simulink library "Pitch_Functions"  (Simulink 6.5)
undefined symbols (not defined in the file or in its folder): A, ABS, B, C, D, P_PitchProfilerAccLim, P_PitchProfilerMaxGain, P_PitchProfilerPostDelay, P_PitchProfilerPreDelay, P_PitchProfilerSpdLim, P_PitchProfilerTc, P_PitchProfilerTcRatio, P_PitchSpinningPos, PITCH_CYCLE_TIME, RND, SQR
libraries: StandardLib x187, WindLib x15, Pitch_Functions x6, simulink x4
(part 1 of 3)
settings Model: Creator=200011716  LastModifiedBy=jschwein

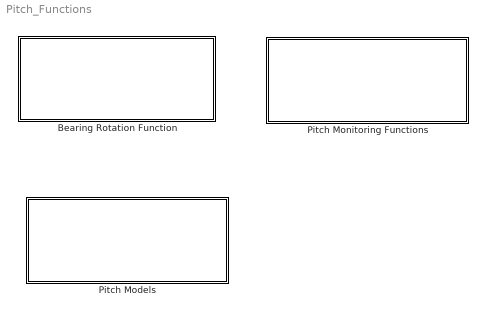
== system Pitch_Functions ==
  Bearing Rotation Function : Subsystem
      mask Display: disp('Bearing Rotation Function (BRF)')
  Pitch Models : Subsystem
      mask Display: disp('Pitch Models')
  Pitch Monitoring Functions : Subsystem
      mask Display: disp('Pitch Monitoring Functions')

== system Pitch_Functions/Bearing Rotation Function ==
  USRB_BladeAtLimSwtchLessthanRef : Subsystem  TreatAsAtomicUnit=on
      settings: MinAlgLoopOccurrences=on
  USRB_BladeAtReferenceDetect : Subsystem  TreatAsAtomicUnit=on
      settings: MinAlgLoopOccurrences=on
  USRB_BladeCompleted : Subsystem  TreatAsAtomicUnit=on
      settings: MinAlgLoopOccurrences=on
  USRB_LimitSwitchPickedUp : Subsystem  TreatAsAtomicUnit=on
      settings: MinAlgLoopOccurrences=on
  USRB_LimitSwitchPickedUpTrail : Subsystem  TreatAsAtomicUnit=on
      settings: MinAlgLoopOccurrences=on
  USRB_StartBladeMotionCmd : Subsystem  TreatAsAtomicUnit=on
      settings: MinAlgLoopOccurrences=on

== system Pitch_Functions/Pitch Models ==
  USRB_PitchProfiler : Subsystem  TreatAsAtomicUnit=on
      settings: MinAlgLoopOccurrences=on

== system Pitch_Functions/Pitch Monitoring Functions ==
  USRB_PitchProfilers : Subsystem  TreatAsAtomicUnit=on
      settings: MinAlgLoopOccurrences=on
  USRB_Pitch_AxisState1 : Subsystem  TreatAsAtomicUnit=on
  USRB_Pitch_BladeImplausible : Subsystem  TreatAsAtomicUnit=on
  USRB_Pitch_BladePitching : Subsystem  TreatAsAtomicUnit=on
  USRB_Pitch_Status : Subsystem  TreatAsAtomicUnit=on
  USRB_SevereBladeProblem : Subsystem  TreatAsAtomicUnit=on
  USRB_TransDelay : Subsystem  TreatAsAtomicUnit=on

== system Pitch_Functions/Bearing Rotation Function/USRB_BladeAtLimSwtchLessthanRef ==
  Limit89Switch : Inport  DataType=boolean
  PitchActual : Inport  Port=2  DataType=single
  Ref : Inport  Port=3  DataType=single
  AND : StandardLib/Logical operations/AND  RepeatCnt=1  SampleTime=-1  ExecutionOrder=0
  Constant : Constant  Value=1  OutDataTypeMode=boolean  OutDataType=sfix(16)  ConRadixGroup=Use specified scaling  OutScaling=2^0  SampleTime=inf  FramePeriod=inf
  Constant1 : Constant  Value=0  OutDataTypeMode=single  OutDataType=sfix(16)  ConRadixGroup=Use specified scaling  OutScaling=2^0  SampleTime=inf  FramePeriod=inf
  LT : StandardLib/Math operations/LT  Equation=<  DataType=SINGLE  SampleTime=-1  ExecutionOrder=0
  MOVE : StandardLib/Memory operations/MOVE  DataType=BOOLEAN  SampleTime=-1  ExecutionOrder=0
  BladeAt89 : Outport  DataType=boolean
  wires:
  Constant1/1 -> LT/3
  Constant/1 -> MOVE/2
  Ref/1 -> LT/2
  MOVE/1 -> AND/1
  LT/1 -> AND/2
  PitchActual/1 -> LT/1
  Limit89Switch/1 -> MOVE/1
  AND/1 -> BladeAt89/1

== system Pitch_Functions/Bearing Rotation Function/USRB_BladeAtReferenceDetect ==
  PitchActual : Inport  DataType=single
  Reference : Inport  Port=2  DataType=single
  PitchSpeed : Inport  Port=3  DataType=single
  PositionSensitivity : Inport  Port=4  DataType=single
  SpeedSensitivity : Inport  Port=5  DataType=single
  FeatherState : Inport  Port=6  DataType=boolean
  AND : StandardLib/Logical operations/AND  RepeatCnt=2  SampleTime=-1  ExecutionOrder=0
  Constant : Constant  Value=0  OutDataTypeMode=single  OutDataType=sfix(16)  ConRadixGroup=Use specified scaling  OutScaling=2^0  SampleTime=inf  FramePeriod=inf
  Constant1 : Constant  Value=0  OutDataTypeMode=single  OutDataType=sfix(16)  ConRadixGroup=Use specified scaling  OutScaling=2^0  SampleTime=inf  FramePeriod=inf
  Constant2 : Constant  Value=0  OutDataTypeMode=single  OutDataType=sfix(16)  ConRadixGroup=Use specified scaling  OutScaling=2^0  SampleTime=inf  FramePeriod=inf
  EQ : StandardLib/Math operations/EQ  Equation===  DataType=SINGLE  SampleTime=-1  ExecutionOrder=0
  EQ1 : StandardLib/Math operations/EQ  Equation===  DataType=SINGLE  SampleTime=-1  ExecutionOrder=0
  BladeAtRef : Outport  DataType=boolean
  wires:
  PitchActual/1 -> EQ/1
  Reference/1 -> EQ/2
  Constant/1 -> EQ/3
  PositionSensitivity/1 -> EQ/4
  PitchSpeed/1 -> EQ1/1
  Constant1/1 -> EQ1/2
  Constant2/1 -> EQ1/3
  SpeedSensitivity/1 -> EQ1/4
  EQ/1 -> AND/1
  EQ1/1 -> AND/2
  AND/1 -> BladeAtRef/1
  FeatherState/1 -> AND/3

== system Pitch_Functions/Bearing Rotation Function/USRB_BladeCompleted ==
  PitchComplete : Inport  DataType=boolean
  PitchActive : Inport  Port=2  DataType=boolean
  BladeAt89 : Inport  Port=3  DataType=boolean
  BRFComplete : Inport  Port=4  DataType=boolean
  ManualReset : Inport  Port=5  DataType=boolean
  LimitSwitch94PickedUp : Inport  Port=6  DataType=boolean
  TooLong : Inport  Port=7  DataType=boolean
  ExtendedPause : Inport  Port=8  DataType=boolean
  Abort : Inport  Port=9  DataType=boolean
  AND : StandardLib/Logical operations/AND  RepeatCnt=1  SampleTime=-1  ExecutionOrder=0
  AND1 : StandardLib/Logical operations/AND  RepeatCnt=1  SampleTime=-1  ExecutionOrder=0
  Constant : Constant  Value=1  OutDataTypeMode=boolean  OutDataType=sfix(16)  ConRadixGroup=Use specified scaling  OutScaling=2^0  SampleTime=inf  FramePeriod=inf
  LATCH : StandardLib/Logical operations/LATCH  SampleTime=-1  ExecutionOrder=0
  OR : StandardLib/Logical operations/OR  RepeatCnt=1  SampleTime=-1  ExecutionOrder=0
  OR1 : StandardLib/Logical operations/OR  RepeatCnt=4  SampleTime=-1  ExecutionOrder=0
  Terminator : Terminator
  BladeComplete : Outport  DataType=boolean
  wires:
  Abort/1 -> OR1/5
  ExtendedPause/1 -> OR1/4
  TooLong/1 -> OR1/3
  PitchActive/1 -> AND/2
  PitchComplete/1 -> AND/1
  Constant/1 -> LATCH/3
  ManualReset/1 -> OR1/2
  BRFComplete/1 -> OR1/1
  OR1/1 -> LATCH/2
  LATCH/2 -> Terminator/1
  LATCH/1 -> BladeComplete/1
  AND1/1 -> OR/2
  BladeAt89/1 -> AND1/1
  OR/1 -> LATCH/1
  LimitSwitch94PickedUp/1 -> AND1/2
  AND/1 -> OR/1

== system Pitch_Functions/Bearing Rotation Function/USRB_LimitSwitchPickedUp ==
  BladeActive : Inport  DataType=boolean
  Limit94Switch1 : Inport  Port=2  DataType=boolean
  Complete : Inport  Port=3  DataType=boolean
  AND : StandardLib/Logical operations/AND  RepeatCnt=1  SampleTime=-1  ExecutionOrder=0
  Constant10 : Constant  Value=1  OutDataTypeMode=boolean  OutDataType=sfix(16)  ConRadixGroup=Use specified scaling  OutScaling=2^0  SampleTime=inf  FramePeriod=inf
  LATCH : StandardLib/Logical operations/LATCH  SampleTime=-1  ExecutionOrder=0
  Terminator12 : Terminator
  LimitSwitchPickedUp : Outport  DataType=boolean
  wires:
  BladeActive/1 -> AND/1
  Limit94Switch1/1 -> AND/2
  AND/1 -> LATCH/1
  Complete/1 -> LATCH/2
  LATCH/1 -> LimitSwitchPickedUp/1
  LATCH/2 -> Terminator12/1
  Constant10/1 -> LATCH/3

== system Pitch_Functions/Bearing Rotation Function/USRB_LimitSwitchPickedUpTrail ==
  BladeActive : Inport  DataType=boolean
  Limit94Switch1 : Inport  Port=2  DataType=boolean
  Complete : Inport  Port=3  DataType=boolean
  AND : StandardLib/Logical operations/AND  RepeatCnt=1  SampleTime=-1  ExecutionOrder=0
  Constant1 : Constant  Value=0  OutDataTypeMode=uint32  OutDataType=sfix(16)  ConRadixGroup=Use specified scaling  OutScaling=2^0  SampleTime=inf  FramePeriod=inf
  Constant10 : Constant  Value=1  OutDataTypeMode=boolean  OutDataType=sfix(16)  ConRadixGroup=Use specified scaling  OutScaling=2^0  SampleTime=inf  FramePeriod=inf
  LATCH : StandardLib/Logical operations/LATCH  SampleTime=-1  ExecutionOrder=0
  NOT : StandardLib/Logical operations/NOT  SampleTime=-1  ExecutionOrder=0
  PULSE1 : StandardLib/Sequencing/PULSE  SampleTime=-1  ExecutionOrder=0
  Terminator{12,14..19} (7 alike) : Terminator
  LimitSwitchPickedUp : Outport  DataType=boolean
  wires:
  PULSE1/1 -> AND/2
  NOT/2 -> PULSE1/1
  Constant1/1 -> PULSE1/2
  PULSE1/6 -> Terminator18/1
  PULSE1/5 -> Terminator17/1
  PULSE1/4 -> Terminator16/1
  PULSE1/3 -> Terminator15/1
  PULSE1/2 -> Terminator14/1
  NOT/1 -> Terminator19/1
  Constant10/1 -> LATCH/3
  LATCH/2 -> Terminator12/1
  LATCH/1 -> LimitSwitchPickedUp/1
  Complete/1 -> LATCH/2
  AND/1 -> LATCH/1
  Limit94Switch1/1 -> NOT/1
  BladeActive/1 -> AND/1

== system Pitch_Functions/Bearing Rotation Function/USRB_StartBladeMotionCmd ==
  Blade_to_Index : Inport  DataType=int16
  bladenum : Inport  Port=2  DataType=int16
  StartCondition : Inport  Port=3  DataType=boolean
  AND : StandardLib/Logical operations/AND  RepeatCnt=1  SampleTime=-1  ExecutionOrder=0
  Constant : Constant  Value=0  OutDataTypeMode=int16  OutDataType=sfix(16)  ConRadixGroup=Use specified scaling  OutScaling=2^0  SampleTime=inf  FramePeriod=inf
  Constant1 : Constant  Value=10000  OutDataTypeMode=uint32  OutDataType=sfix(16)  ConRadixGroup=Use specified scaling  OutScaling=2^0  SampleTime=inf  FramePeriod=inf
  EQ : StandardLib/Math operations/EQ  Equation===  DataType=INT16  SampleTime=-1  ExecutionOrder=0
  PULSE : StandardLib/Sequencing/PULSE  SampleTime=-1  ExecutionOrder=0
  Terminator{,1..4} (5 alike) : Terminator
  StartBlade : Outport  DataType=boolean
  wires:
  Constant1/1 -> PULSE/2
  PULSE/6 -> Terminator4/1
  PULSE/5 -> Terminator3/1
  PULSE/4 -> Terminator2/1
  PULSE/3 -> Terminator1/1
  PULSE/2 -> Terminator/1
  PULSE/1 -> StartBlade/1
  StartCondition/1 -> AND/2
  AND/1 -> PULSE/1
  bladenum/1 -> EQ/2
  Blade_to_Index/1 -> EQ/1
  EQ/1 -> AND/1
  Constant/1 -> EQ/4, EQ/3

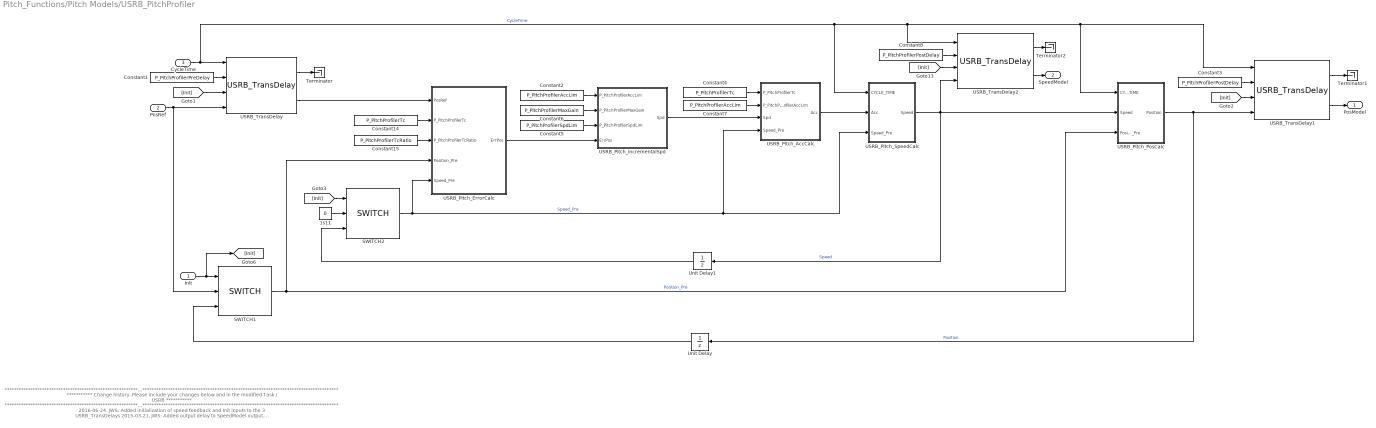
== system Pitch_Functions/Pitch Models/USRB_PitchProfiler ==
  note: ***********************************************************************************************************************************************
      | ***********         Change history. Please include your changes below and in the modified Task / USRB         ***********
      | ***********************************************************************************************************************************************
      | 2016-06-24, JWS: Added initialization of speed feedback and Init inputs to the 3 USRB_TransDelays
      | 2015-03-21, JWS: Added output delay to SpeedModel output.
      | 2015-11-04, JWS: Updated USRB name.
      | 2015-09-11, JWS: Replaced constant blocks with inputs.  Added SpeedModel output.
      | ***********************************************************************************************************************************************
  Init : Inport  DataType=boolean
  PosRef : Inport  Port=2  DataType=single
  CycleTime : Inport  Port=3  DataType=single
  1s11 : Constant  Value=0  OutDataTypeMode=single  OutDataType=sfix(16)  ConRadixGroup=Use specified scaling  OutScaling=2^0  SampleTime=inf  FramePeriod=inf
  Constant1 : Constant  Value=P_PitchProfilerPreDelay  OutDataTypeMode=uint32  OutDataType=sfix(16)  ConRadixGroup=Use specified scaling  OutScaling=2^0  SampleTime=-1  FramePeriod=inf
  Constant14 : Constant  Value=P_PitchProfilerTc  OutDataTypeMode=single  OutDataType=sfix(16)  ConRadixGroup=Use specified scaling  OutScaling=2^0  SampleTime=-1  FramePeriod=inf
  Constant15 : Constant  Value=P_PitchProfilerTcRatio  OutDataTypeMode=single  OutDataType=sfix(16)  ConRadixGroup=Use specified scaling  OutScaling=2^0  SampleTime=-1  FramePeriod=inf
  Constant2 : Constant  Value=P_PitchProfilerAccLim  OutDataTypeMode=single  OutDataType=sfix(16)  ConRadixGroup=Use specified scaling  OutScaling=2^0  SampleTime=-1  FramePeriod=inf
  Constant3 : Constant  Value=P_PitchProfilerPostDelay  OutDataTypeMode=uint32  OutDataType=sfix(16)  ConRadixGroup=Use specified scaling  OutScaling=2^0  SampleTime=-1  FramePeriod=inf
  Constant4 : Constant  Value=P_PitchProfilerTc  OutDataTypeMode=single  OutDataType=sfix(16)  ConRadixGroup=Use specified scaling  OutScaling=2^0  SampleTime=-1  FramePeriod=inf
  Constant5 : Constant  Value=P_PitchProfilerSpdLim  OutDataTypeMode=single  OutDataType=sfix(16)  ConRadixGroup=Use specified scaling  OutScaling=2^0  SampleTime=-1  FramePeriod=inf
  Constant6 : Constant  Value=P_PitchProfilerMaxGain  OutDataTypeMode=single  OutDataType=sfix(16)  ConRadixGroup=Use specified scaling  OutScaling=2^0  SampleTime=-1  FramePeriod=inf
  Constant7 : Constant  Value=P_PitchProfilerAccLim  OutDataTypeMode=single  OutDataType=sfix(16)  ConRadixGroup=Use specified scaling  OutScaling=2^0  SampleTime=-1  FramePeriod=inf
  Constant8 : Constant  Value=P_PitchProfilerPostDelay  OutDataTypeMode=uint32  OutDataType=sfix(16)  ConRadixGroup=Use specified scaling  OutScaling=2^0  SampleTime=-1  FramePeriod=inf
  SWITCH1 : StandardLib/Memory operations/SWITCH  DataType=SINGLE  SampleTime=-1  ExecutionOrder=0
  SWITCH2 : StandardLib/Memory operations/SWITCH  DataType=SINGLE  SampleTime=-1  ExecutionOrder=0
  Terminator : Terminator
  Terminator1 : Terminator
  Terminator2 : Terminator
  USRB_Pitch_AccCalc : Subsystem  TreatAsAtomicUnit=on
  USRB_Pitch_ErrorCalc : Subsystem  TreatAsAtomicUnit=on
  USRB_Pitch_IncrementalSpd : Subsystem  TreatAsAtomicUnit=on
  USRB_Pitch_PosCalc : Subsystem  TreatAsAtomicUnit=on
  USRB_Pitch_SpeedCalc : Subsystem  TreatAsAtomicUnit=on
  USRB_TransDelay : Pitch_Functions/Pitch Monitoring Functions/USRB_TransDelay  SystemSampleTime=-1
  USRB_TransDelay1 : Pitch_Functions/Pitch Monitoring Functions/USRB_TransDelay  SystemSampleTime=-1
  USRB_TransDelay2 : Pitch_Functions/Pitch Monitoring Functions/USRB_TransDelay  SystemSampleTime=-1
  Unit Delay : UnitDelay  Orientation=left  SampleTime=-1
  Unit Delay1 : UnitDelay  Orientation=left  SampleTime=-1
  PosModel : Outport  DataType=single
  SpeedModel : Outport  Port=2  DataType=single
  wires:
  USRB_TransDelay1/2 -> PosModel/1
  Init/1 -> SWITCH1/1, [Init]
  Unit Delay/1 -> SWITCH1/3
  USRB_Pitch_SpeedCalc/1(Speed) -> USRB_Pitch_PosCalc/2(Speed), Unit Delay1/1, USRB_TransDelay2/4  "Speed"
  USRB_Pitch_AccCalc/1(Acc) -> USRB_Pitch_SpeedCalc/2(Acc)
  USRB_Pitch_IncrementalSpd/1(Spd) -> USRB_Pitch_AccCalc/3(Spd)
  USRB_Pitch_ErrorCalc/1(ErrPos) -> USRB_Pitch_IncrementalSpd/4(ErrPos)
  SWITCH1/1 -> USRB_Pitch_PosCalc/3(Position_Pre), USRB_Pitch_ErrorCalc/4(Position_Pre)  "Position_Pre"
  USRB_TransDelay/2 -> USRB_Pitch_ErrorCalc/1(PosRef)
  USRB_Pitch_PosCalc/1(Position) -> Unit Delay/1, USRB_TransDelay1/4  "Position"
  Constant1/1 -> USRB_TransDelay/2
  USRB_TransDelay/1 -> Terminator/1
  USRB_TransDelay1/1 -> Terminator1/1
  CycleTime/1 -> USRB_TransDelay/1, USRB_Pitch_SpeedCalc/1(CYCLE_TIME), USRB_Pitch_PosCalc/1(CYCLE_TIME), USRB_TransDelay1/1, USRB_TransDelay2/1  "CycleTime"
  Constant14/1 -> USRB_Pitch_ErrorCalc/2(P_PitchProfilerTc)
  Constant15/1 -> USRB_Pitch_ErrorCalc/3(P_PitchProfilerTcRatio)
  Constant2/1 -> USRB_Pitch_IncrementalSpd/1(P_PitchProfilerAccLim)
  Constant6/1 -> USRB_Pitch_IncrementalSpd/2(P_PitchProfilerMaxGain)
  Constant5/1 -> USRB_Pitch_IncrementalSpd/3(P_PitchProfilerSpdLim)
  Constant3/1 -> USRB_TransDelay1/2
  Constant4/1 -> USRB_Pitch_AccCalc/1(P_PitchProfilerTc)
  Constant7/1 -> USRB_Pitch_AccCalc/2(P_PitchProfilerAccLim)
  Constant8/1 -> USRB_TransDelay2/2
  USRB_TransDelay2/1 -> Terminator2/1
  USRB_TransDelay2/2 -> SpeedModel/1
  PosRef/1 -> USRB_TransDelay/4, SWITCH1/2
  [Init] -> USRB_TransDelay/3
  [Init] -> USRB_TransDelay2/3
  [Init] -> USRB_TransDelay1/3
  [Init] -> SWITCH2/1
  1s11/1 -> SWITCH2/2
  SWITCH2/1 -> USRB_Pitch_ErrorCalc/5(Speed_Pre), USRB_Pitch_AccCalc/4(Speed_Pre), USRB_Pitch_SpeedCalc/3(Speed_Pre)  "Speed_Pre"
  Unit Delay1/1 -> SWITCH2/3

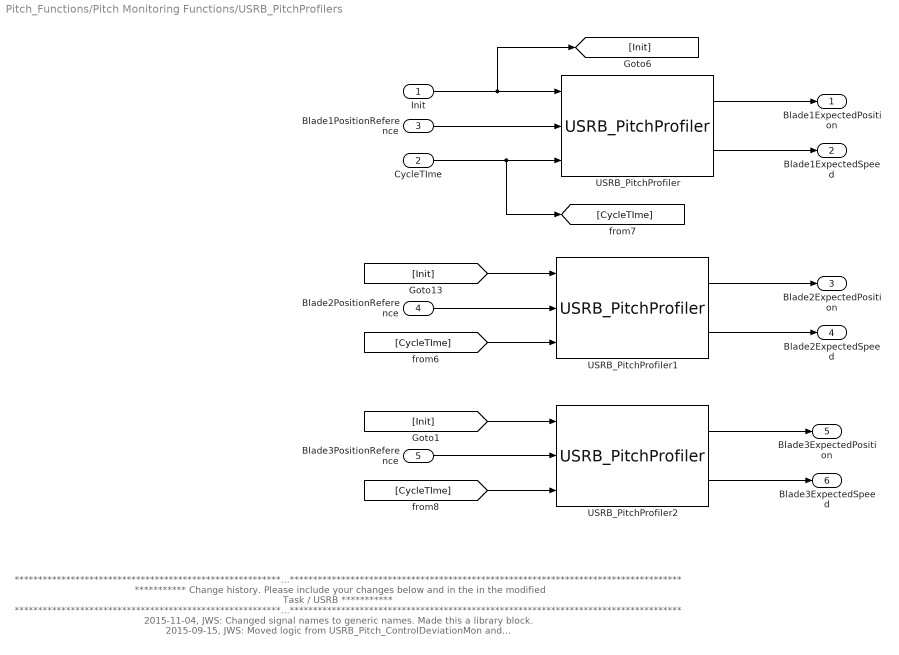
== system Pitch_Functions/Pitch Monitoring Functions/USRB_PitchProfilers ==
  note: ***********************************************************************************************************************************************
      | ***********         Change history. Please include your changes below and in the in the modified Task / USRB         ***********
      | ***********************************************************************************************************************************************
      | 2015-11-04, JWS: Changed signal names to generic names.  Made this a library block.
      | 2015-09-15, JWS: Moved logic from USRB_Pitch_ControlDeviationMon and USRB_Pitch_BladeAngleAsymMon.  Updated
      |                               initialization logic.
  Init : Inport  DataType=boolean
  CycleTIme : Inport  Port=2  DataType=single
  Blade1PositionReference : Inport  Port=3  DataType=single
  Blade2PositionReference : Inport  Port=4  DataType=single
  Blade3PositionReference : Inport  Port=5  DataType=single
  USRB_PitchProfiler : Pitch_Functions/Pitch Models/USRB_PitchProfiler  SystemSampleTime=-1
  USRB_PitchProfiler1 : Pitch_Functions/Pitch Models/USRB_PitchProfiler  SystemSampleTime=-1
  USRB_PitchProfiler2 : Pitch_Functions/Pitch Models/USRB_PitchProfiler  SystemSampleTime=-1
  Blade1ExpectedPosition : Outport  DataType=single
  Blade1ExpectedSpeed : Outport  Port=2  DataType=single
  Blade2ExpectedPosition : Outport  Port=3  DataType=single
  Blade2ExpectedSpeed : Outport  Port=4  DataType=single
  Blade3ExpectedPosition : Outport  Port=5  DataType=single
  Blade3ExpectedSpeed : Outport  Port=6  DataType=single
  wires:
  [CycleTIme] -> USRB_PitchProfiler2/3
  [CycleTIme] -> USRB_PitchProfiler1/3
  CycleTIme/1 -> [CycleTIme], USRB_PitchProfiler/3
  USRB_PitchProfiler2/2 -> Blade3ExpectedSpeed/1
  USRB_PitchProfiler2/1 -> Blade3ExpectedPosition/1
  USRB_PitchProfiler1/2 -> Blade2ExpectedSpeed/1
  USRB_PitchProfiler1/1 -> Blade2ExpectedPosition/1
  [Init] -> USRB_PitchProfiler1/1
  [Init] -> USRB_PitchProfiler2/1
  Blade2PositionReference/1 -> USRB_PitchProfiler1/2
  Blade3PositionReference/1 -> USRB_PitchProfiler2/2
  USRB_PitchProfiler/2 -> Blade1ExpectedSpeed/1
  USRB_PitchProfiler/1 -> Blade1ExpectedPosition/1
  Init/1 -> [Init], USRB_PitchProfiler/1
  Blade1PositionReference/1 -> USRB_PitchProfiler/2
